simulink model "MATLAB_TEST"  (R2019b)
settings: Solver=FixedStepDiscrete  StartTime=0  StopTime=50  FixedStep=0.0025  RelTol=1e-3
undefined symbols (not defined in the file): BCM_COM_PROC_P20, BCM_COM_PROC_P20_SFW_R2018b, BCM_COM_PROC_P2_5, BCM_COM_PROC_P2_5_SFW_R2018b, BCM_COM_PROC_P5, BCM_COM_PROC_P5_SFW_R2018b, BCMA_ACCU_PT_Conf_Flt, BCMA_ACCU_PT_Unconf_Flt, BCMA_Antiskid_Off_Sanction, BCMA_Avionics_Conf_Flt, BCMA_BCM_CCDL_Conf_Flt, BCMA_BCM_CCDL_Unconf_Flt, BCMA_BCM_DBCU_INHIBITION_Conf_Flt, BCMA_BCM_DBCU_INHIBITION_Unconf_Flt, BCMA_BCP_ALT_Disp_Sw_Conf_Flt, BCMA_BCP_ALT_Disp_Sw_Unconf_Flt, BCMA_BCP_ALT_SW_ON_CMD_Conf_Flt, BCMA_BCP_ALT_SW_ON_CMD_Unconf_Flt, BCMA_BCP_PARK_OFF_SW_CMD_Conf_Flt, BCMA_BCP_PARK_OFF_SW_CMD_Unconf_Flt, BCMA_CF_BSELV_JCL, BCMA_CF_BSELV_JOP, BCMA_CF_BSELV_OC, BCMA_CF_BSELV_SC, BCMA_CF_LH_SV_JCL, BCMA_CF_LH_SV_JOP, BCMA_CF_LH_SV_OC, BCMA_CF_LH_SV_SC, BCMA_CF_PARK_BRK, BCMA_CF_RESIDUAL_PRESS, BCMA_CF_RH_SV_JCL, BCMA_CF_RH_SV_JOP, BCMA_CF_RH_SV_OC, BCMA_CF_RH_SV_SC, BCMA_CF_SELV_JCL, BCMA_CF_SELV_JOP, BCMA_CF_SELV_OC, BCMA_CF_SELV_SC, BCMA_CF_SV_DRIFT, BCMA_DBCU_ALT_MODE_Conf_Flt, BCMA_DBCU_ALT_MODE_Unconf_Flt, BCMA_DBCU_BRK_ORDER_FAIL_Conf_Flt, BCMA_DBCU_BRK_ORDER_FAIL_Unconf_Flt, BCMA_DBCU_Conf_Flt, BCMA_DBCU_DISPATCH_SW_ON_Conf_Flt, BCMA_DBCU_DISPATCH_SW_ON_Unconf_Flt, BCMA_DBCU_FAILED_Conf_Flt, BCMA_DBCU_FAILED_Unconf_Flt, BCMA_DFCS1_Capsule_Validity, BCMA_DFCS1_Label202_Corrupted, BCMA_DFCS1_Label202_Not_Refreshed, BCMA_DFCS1_Label204_Corrupted, BCMA_DFCS1_Label204_Not_Refreshed, BCMA_DFCS1_Label205_Corrupted, BCMA_DFCS1_Label205_Not_Refreshed, BCMA_DFCS1_Label206_Corrupted, BCMA_DFCS1_Label206_Not_Refreshed, BCMA_DFCS1_Label207_Corrupted, BCMA_DFCS1_Label207_Not_Refreshed, BCMA_DFCS3_Capsule_Validity ... (+762)
libraries: simulink x73, lib_MBD_Control x5
(part 16 of 16)

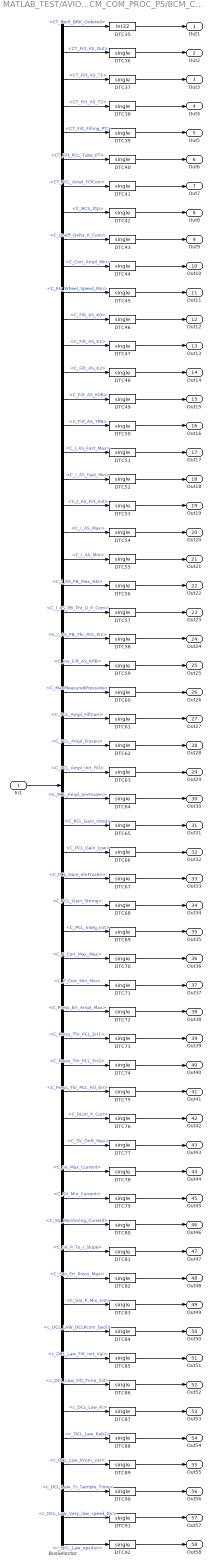
== system MATLAB_TEST/AVIONICS/Brake_Control_Module_Side_A/BCSA Controller CP/BCM_COM_PROC_P5/BCM_COM_PROC_P5/Subsystem ==
  In1 : Inport
  BusSelector : BusSelector  OutputSignals=CT_Conf_BRK_Ordered,CT_Filt_AS_Out,CT_Filt_AS_T1,CT_Filt_AS_T2,CT_Filt_Filling_PT,CT_Filt_PCL_Tube_PT,CT_PCL_Ampl_FillCorr,C_BCS_Ztp,C_Coeff_Delta_P_Com,C_Corr_Ampl_Min,C_Err_Wheel_Speed_Min,C_Filt_AS_K0,C_Filt_AS_K1,C_Filt_AS_K2,C_Filt_AS_KPB,C_Filt_AS_TPB,C_I_AS_Fast_Max,C_I_AS_Fast_Min,C_I_AS_Filt_Init,C_I_AS_Max,C_I_AS_Min,C_I_AS_PB_Max_ND,C_I_AS_PB_Thr_D_P_Com,C_I_AS_PB_Thr_PCL_Frz,C_Inv_Filt_AS_KPB,C_MaxMeasuredPressure,C_PCL_Ampl_FillCorr,C_PCL_Ampl_Frozen,C_PCL_Ampl_Init_Fill,C_PCL_Ampl_SmFrozen,C_PCL_Gain_Integ,C_PCL_Gain_Low,C_PCL_Gain_SmFrozen,C_PCL_Gain_Strong,C_PCL_Integ_Init,C_P_Corr_Max_Max,C_P_Corr_Min_Min,C_Press_Err_Ampl_Max,C_Press_Thr_PCL_Err1,C_Press_Thr_PCL_Err2,C_Press_Thr_PCL_Fill_Err,C_RLim_P_Corr,C_SV_Drift_Max,C_SV_Max_Current,C_SV_Min_Current,C_SV_Monitoring_Current,C_SV_P_To_I_Slope,C_Squ_Err_Press_Max,C_Val_P_Min_Init,c_DCL_LAW_DCLPcom_bool,c_DCL_Law_Filt_Init_Val,c_DCL_Law_Filt_Time_Cst,c_DCL_Law_Ki,c_DCL_Law_Kpb2,c_DCL_Law_Pcom_var,c_DCL_Law_Ts_Sample_Time,c_DCL_Law_Very_law_speed_thr,c_DCL_Law_epsilon
  DTC35 : DataTypeConversion  OutDataTypeStr=int32  SaturateOnIntegerOverflow=on  RndMeth=Zero
  DTC{36..92} (57 alike) : DataTypeConversion  OutDataTypeStr=single  SaturateOnIntegerOverflow=on  RndMeth=Zero
  Out1 : Outport
  Out2 : Outport  Port=2
  Out3 : Outport  Port=3
  Out4 : Outport  Port=4
  Out5 : Outport  Port=5
  Out6 : Outport  Port=6
  Out7 : Outport  Port=7
  Out8 : Outport  Port=8
  Out9 : Outport  Port=9
  Out10 : Outport  Port=10
  Out11 : Outport  Port=11
  Out12 : Outport  Port=12
  Out13 : Outport  Port=13
  Out14 : Outport  Port=14
  Out15 : Outport  Port=15
  Out16 : Outport  Port=16
  Out17 : Outport  Port=17
  Out18 : Outport  Port=18
  Out19 : Outport  Port=19
  Out20 : Outport  Port=20
  Out21 : Outport  Port=21
  Out22 : Outport  Port=22
  Out23 : Outport  Port=23
  Out24 : Outport  Port=24
  Out25 : Outport  Port=25
  Out26 : Outport  Port=26
  Out27 : Outport  Port=27
  Out28 : Outport  Port=28
  Out29 : Outport  Port=29
  Out30 : Outport  Port=30
  Out31 : Outport  Port=31
  Out32 : Outport  Port=32
  Out33 : Outport  Port=33
  Out34 : Outport  Port=34
  Out35 : Outport  Port=35
  Out36 : Outport  Port=36
  Out37 : Outport  Port=37
  Out38 : Outport  Port=38
  Out39 : Outport  Port=39
  Out40 : Outport  Port=40
  Out41 : Outport  Port=41
  Out42 : Outport  Port=42
  Out43 : Outport  Port=43
  Out44 : Outport  Port=44
  Out45 : Outport  Port=45
  Out46 : Outport  Port=46
  Out47 : Outport  Port=47
  Out48 : Outport  Port=48
  Out49 : Outport  Port=49
  Out50 : Outport  Port=50
  Out51 : Outport  Port=51
  Out52 : Outport  Port=52
  Out53 : Outport  Port=53
  Out54 : Outport  Port=54
  Out55 : Outport  Port=55
  Out56 : Outport  Port=56
  Out57 : Outport  Port=57
  Out58 : Outport  Port=58
  wires:
  BusSelector/45 -> DTC79/1  "<C_SV_Min_Current>"
  BusSelector/40 -> DTC74/1  "<C_Press_Thr_PCL_Err2>"
  BusSelector/20 -> DTC54/1  "<C_I_AS_Max>"
  DTC48/1 -> Out14/1
  DTC79/1 -> Out45/1
  In1/1 -> BusSelector/1
  BusSelector/51 -> DTC85/1  "<c_DCL_Law_Filt_Init_Val>"
  BusSelector/21 -> DTC55/1  "<C_I_AS_Min>"
  BusSelector/14 -> DTC48/1  "<C_Filt_AS_K2>"
  BusSelector/7 -> DTC41/1  "<CT_PCL_Ampl_FillCorr>"
  BusSelector/15 -> DTC49/1  "<C_Filt_AS_KPB>"
  BusSelector/27 -> DTC61/1  "<C_PCL_Ampl_FillCorr>"
  BusSelector/3 -> DTC37/1  "<CT_Filt_AS_T1>"
  BusSelector/12 -> DTC46/1  "<C_Filt_AS_K0>"
  BusSelector/58 -> DTC92/1  "<c_DCL_Law_epsilon>"
  BusSelector/19 -> DTC53/1  "<C_I_AS_Filt_Init>"
  BusSelector/1 -> DTC35/1  "<CT_Conf_BRK_Ordered>"
  BusSelector/32 -> DTC66/1  "<C_PCL_Gain_Low>"
  DTC52/1 -> Out18/1
  BusSelector/25 -> DTC59/1  "<C_Inv_Filt_AS_KPB>"
  DTC63/1 -> Out29/1
  BusSelector/8 -> DTC42/1  "<C_BCS_Ztp>"
  BusSelector/36 -> DTC70/1  "<C_P_Corr_Max_Max>"
  BusSelector/4 -> DTC38/1  "<CT_Filt_AS_T2>"
  BusSelector/55 -> DTC89/1  "<c_DCL_Law_Pcom_var>"
  DTC73/1 -> Out39/1
  BusSelector/10 -> DTC44/1  "<C_Corr_Ampl_Min>"
  BusSelector/5 -> DTC39/1  "<CT_Filt_Filling_PT>"
  BusSelector/48 -> DTC82/1  "<C_Squ_Err_Press_Max>"
  BusSelector/18 -> DTC52/1  "<C_I_AS_Fast_Min>"
  BusSelector/31 -> DTC65/1  "<C_PCL_Gain_Integ>"
  BusSelector/39 -> DTC73/1  "<C_Press_Thr_PCL_Err1>"
  BusSelector/17 -> DTC51/1  "<C_I_AS_Fast_Max>"
  BusSelector/9 -> DTC43/1  "<C_Coeff_Delta_P_Com>"
  BusSelector/34 -> DTC68/1  "<C_PCL_Gain_Strong>"
  BusSelector/24 -> DTC58/1  "<C_I_AS_PB_Thr_PCL_Frz>"
  BusSelector/30 -> DTC64/1  "<C_PCL_Ampl_SmFrozen>"
  BusSelector/57 -> DTC91/1  "<c_DCL_Law_Very_law_speed_thr>"
  BusSelector/2 -> DTC36/1  "<CT_Filt_AS_Out>"
  BusSelector/44 -> DTC78/1  "<C_SV_Max_Current>"
  BusSelector/42 -> DTC76/1  "<C_RLim_P_Corr>"
  BusSelector/16 -> DTC50/1  "<C_Filt_AS_TPB>"
  BusSelector/38 -> DTC72/1  "<C_Press_Err_Ampl_Max>"
  BusSelector/46 -> DTC80/1  "<C_SV_Monitoring_Current>"
  BusSelector/54 -> DTC88/1  "<c_DCL_Law_Kpb2>"
  BusSelector/26 -> DTC60/1  "<C_MaxMeasuredPressure>"
  BusSelector/6 -> DTC40/1  "<CT_Filt_PCL_Tube_PT>"
  BusSelector/29 -> DTC63/1  "<C_PCL_Ampl_Init_Fill>"
  DTC43/1 -> Out9/1
  BusSelector/11 -> DTC45/1  "<C_Err_Wheel_Speed_Min>"
  BusSelector/56 -> DTC90/1  "<c_DCL_Law_Ts_Sample_Time>"
  BusSelector/37 -> DTC71/1  "<C_P_Corr_Min_Min>"
  DTC62/1 -> Out28/1
  BusSelector/47 -> DTC81/1  "<C_SV_P_To_I_Slope>"
  DTC80/1 -> Out46/1
  BusSelector/52 -> DTC86/1  "<c_DCL_Law_Filt_Time_Cst>"
  BusSelector/41 -> DTC75/1  "<C_Press_Thr_PCL_Fill_Err>"
  BusSelector/22 -> DTC56/1  "<C_I_AS_PB_Max_ND>"
  BusSelector/43 -> DTC77/1  "<C_SV_Drift_Max>"
  BusSelector/53 -> DTC87/1  "<c_DCL_Law_Ki>"
  BusSelector/35 -> DTC69/1  "<C_PCL_Integ_Init>"
  BusSelector/33 -> DTC67/1  "<C_PCL_Gain_SmFrozen>"
  DTC67/1 -> Out33/1
  BusSelector/50 -> DTC84/1  "<c_DCL_LAW_DCLPcom_bool>"
  BusSelector/28 -> DTC62/1  "<C_PCL_Ampl_Frozen>"
  BusSelector/23 -> DTC57/1  "<C_I_AS_PB_Thr_D_P_Com>"
  BusSelector/13 -> DTC47/1  "<C_Filt_AS_K1>"
  DTC56/1 -> Out22/1
  BusSelector/49 -> DTC83/1  "<C_Val_P_Min_Init>"
  DTC74/1 -> Out40/1
  DTC82/1 -> Out48/1
  DTC65/1 -> Out31/1
  DTC78/1 -> Out44/1
  DTC70/1 -> Out36/1
  DTC35/1 -> Out1/1
  DTC75/1 -> Out41/1
  DTC76/1 -> Out42/1
  DTC42/1 -> Out8/1
  DTC44/1 -> Out10/1
  DTC45/1 -> Out11/1
  DTC40/1 -> Out6/1
  DTC38/1 -> Out4/1
  DTC84/1 -> Out50/1
  DTC39/1 -> Out5/1
  DTC37/1 -> Out3/1
  DTC61/1 -> Out27/1
  DTC64/1 -> Out30/1
  DTC36/1 -> Out2/1
  DTC72/1 -> Out38/1
  DTC85/1 -> Out51/1
  DTC55/1 -> Out21/1
  DTC59/1 -> Out25/1
  DTC41/1 -> Out7/1
  DTC83/1 -> Out49/1
  DTC47/1 -> Out13/1
  DTC92/1 -> Out58/1
  DTC89/1 -> Out55/1
  DTC88/1 -> Out54/1
  DTC53/1 -> Out19/1
  DTC86/1 -> Out52/1
  DTC91/1 -> Out57/1
  DTC87/1 -> Out53/1
  DTC77/1 -> Out43/1
  DTC71/1 -> Out37/1
  DTC69/1 -> Out35/1
  DTC68/1 -> Out34/1
  DTC66/1 -> Out32/1
  DTC58/1 -> Out24/1
  DTC81/1 -> Out47/1
  DTC60/1 -> Out26/1
  DTC57/1 -> Out23/1
  DTC50/1 -> Out16/1
  DTC51/1 -> Out17/1
  DTC90/1 -> Out56/1
  DTC49/1 -> Out15/1
  DTC46/1 -> Out12/1
  DTC54/1 -> Out20/1
